simulink model "Parafoil_NL_6DoF_with_Guidance"  (R2019a)
settings: Solver=VariableStepAuto  StartTime=0.0  StopTime=400  RelTol=1e-3
values from neighbouring files (symbols this model uses):
  b = 1.8    [Parafoil_init.m]    (also in Parafoil_init_with_guidance.m)
  c = 3    [Nico_PhaseIIController.m]    (also in Parafoil_init.m = 0.75; Parafoil_init_with_guidance.m = 0.75)
  CD_0 = .153    (= 0.153)    [Parafoil_init.m]    (also in Parafoil_init_with_guidance.m)
  CD_a2 = 2.4    [Parafoil_init.m]    (also in Parafoil_init_with_guidance.m)
  CD_db = .043    (= 0.043)    [Parafoil_init.m]    (also in Parafoil_init_with_guidance.m)
  CD_p = .5    (= 0.5)    [Parafoil_init.m]    (also in Parafoil_init_with_guidance.m)
  CL_0 = 0    [Parafoil_init.m]    (also in Parafoil_init_with_guidance.m)
  CL_a = 3.9    [Parafoil_init.m]    (also in Parafoil_init_with_guidance.m)
  CL_a2db = 2.062    [Parafoil_init.m]    (also in Parafoil_init_with_guidance.m)
  CL_a3 = 20    [Parafoil_init.m]    (also in Parafoil_init_with_guidance.m)
  CL_adb = .39    (= 0.39)    [Parafoil_init.m]    (also in Parafoil_init_with_guidance.m)
  Cl_b = .001    (= 0.001)    [Parafoil_init.m]    (also in Parafoil_init_with_guidance.m)
  Cl_da = 0    [Parafoil_init.m]    (also in Parafoil_init_with_guidance.m)
  CL_db = 0    [Parafoil_init.m]    (also in Parafoil_init_with_guidance.m)
  Cl_p = -.1    (= -0.1)    [Parafoil_init.m]    (also in Parafoil_init_with_guidance.m)
  Cl_r = 0    [Parafoil_init.m]    (also in Parafoil_init_with_guidance.m)
  Cm_db = 0    [Parafoil_init.m]    (also in Parafoil_init_with_guidance.m)
  Cm_q = -2.5    [Parafoil_init.m]    (also in Parafoil_init_with_guidance.m)
  Cn_b = .02    (= 0.02)    [Parafoil_init.m]    (also in Parafoil_init_with_guidance.m)
  Cn_da = .005    (= 0.005)    [Parafoil_init.m]    (also in Parafoil_init_with_guidance.m)
  Cn_da2 = 0    [Parafoil_init.m]    (also in Parafoil_init_with_guidance.m)
  Cn_p = 0    [Parafoil_init.m]    (also in Parafoil_init_with_guidance.m)
  Cn_r = -.11    (= -0.11)    [Parafoil_init.m]    (also in Parafoil_init_with_guidance.m)
  CY_b = -1    [Parafoil_init.m]    (also in Parafoil_init_with_guidance.m)
  db = 0.5*(delR+delL)    (= 0.5)    [Parafoil_init.m]    (also in Parafoil_init_with_guidance.m)
  g = 9.81    [Parafoil_init.m]    (also in Parafoil_init_with_guidance.m)
  gamma_0 = -25*pi/180    (= -0.436332312999)    [Parafoil_init.m]    (also in Parafoil_init_with_guidance.m)
  I_AI = diag([.07 .06 .046])    [Parafoil_init.m]    (also in Parafoil_init_with_guidance.m)
  I_AM = diag([.05 .35 1.85])    [Parafoil_init.m]    (also in Parafoil_init_with_guidance.m)
  I_B = [Ixx Ixy Ixz ... (first row only)    [Parafoil_init.m]    (also in Parafoil_init_with_guidance.m)
  Kd = 0.001    [ARES_GNC_V006_2D.m]    (also in ARES_GNC_V009_2D.m; ARES_GNC_V009_2D_MultiPLot.m; Nico_PhaseIIController.m = 0.5; Parafoil_init_with_guidance.m = 0)
  Ki = 0.003    [ARES_GNC_V006_2D.m]    (also in ARES_GNC_V009_2D.m; ARES_GNC_V009_2D_MultiPLot.m; Nico_PhaseIIController.m = 0.1; Parafoil_init_with_guidance.m = 0.0009)
  Kp = 0.90    (= 0.9)    [ARES_GNC_V006_2D.m]    (also in ARES_GNC_V009_2D.m = 0.05; ARES_GNC_V009_2D_MultiPLot.m = 0.05; Nico_PhaseIIController.m; Parafoil_init_with_guidance.m = 1)
  m = 2.7    [Parafoil_init.m]    (also in Parafoil_init_with_guidance.m)
  p_h = [30;25;0]    [Parafoil_init_with_guidance.m]
  phi_0 = 0*pi/180    (= 0)    [Parafoil_init.m]    (also in Parafoil_init_with_guidance.m)
  psi_0 = 0    [Parafoil_init.m]    (also in Parafoil_init_with_guidance.m)
  r_cg2c = [.5;0;-4]    [Parafoil_init.m]    (also in Parafoil_init_with_guidance.m)
  r_cg2p = [-2; 0; 1]    [Parafoil_init.m]    (also in Parafoil_init_with_guidance.m)
  rho = 1.3    [Parafoil_init.m]    (also in Parafoil_init_with_guidance.m)
  S_rcg2c = [0 -r_cg2c(3) r_cg2c(2) ... (first row only)    [Parafoil_init.m]    (also in Parafoil_init_with_guidance.m)
  Sc = b*c    (= 1.35)    [Parafoil_init.m]    (also in Parafoil_init_with_guidance.m)
  Sp = .01    (= 0.01)    [Parafoil_init.m]    (also in Parafoil_init_with_guidance.m)
  theta_0 = 0*pi/180    (= 0)    [Parafoil_init.m]    (also in Parafoil_init_with_guidance.m)
  v_0 = [7.135; 0; 4.222]    [Parafoil_init.m]    (also in Parafoil_init_with_guidance.m)
  Vw_x = 0    [Parafoil_init.m]    (also in Parafoil_init_with_guidance.m)
  Vw_y = 0    [Parafoil_init.m]    (also in Parafoil_init_with_guidance.m)
  Vw_z = 0    [Parafoil_init.m]    (also in Parafoil_init_with_guidance.m)
  w_0 = [0;0;0]    [Parafoil_init.m]    (also in Parafoil_init_with_guidance.m)
libraries: vrlib x7, simulink x1
settings Model: Creator=chengl2  LastModifiedBy=curryn

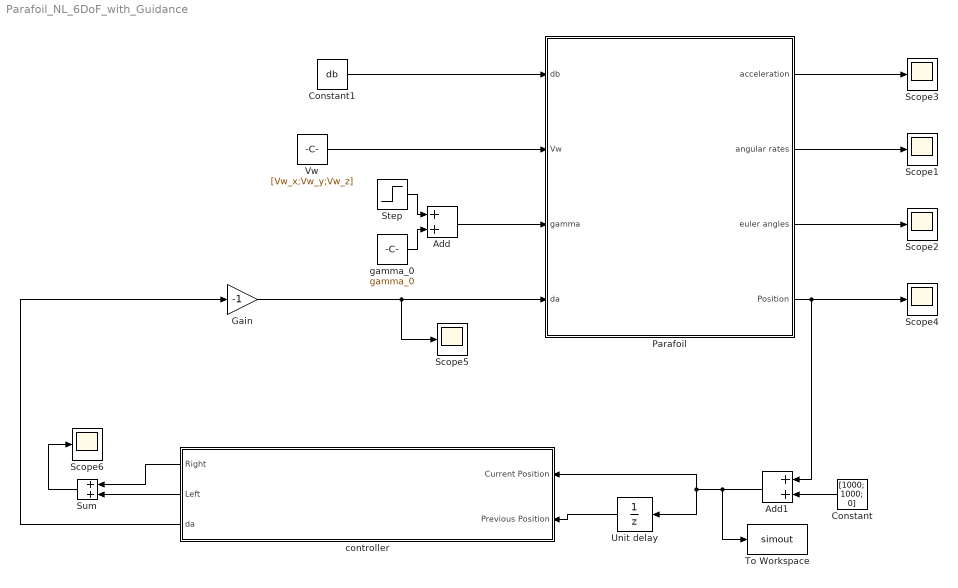
== system Parafoil_NL_6DoF_with_Guidance ==
  Add : Sum
  Add1 : Sum
  Constant : Constant  Value=[1000; 1000; 0]
  Constant1 : Constant  Value=db
  Gain : Gain  Gain=-1
  Parafoil : Subsystem
  Scope{1..6} (6 alike) : Scope
  Step : Step  Time=10  After=0*pi/180  SampleTime=0
  Sum : Sum
  To Workspace : ToWorkspace  VariableName=simout  SaveFormat=Timeseries  SampleTime=-1
  Unit delay : UnitDelay  SampleTime=-1  HasFrameUpgradeWarning=on
  Vw : Constant  Value=[Vw_x;Vw_y;Vw_z]  VectorParams1D=off
  controller : Subsystem
  gamma_0 : Constant  Value=gamma_0
  wires:
  gamma_0/1 -> Add/2
  Step/1 -> Add/1
  Vw/1 -> Parafoil/2(Vw)
  Add/1 -> Parafoil/3(gamma)
  Parafoil/1(acceleration) -> Scope3/1
  Parafoil/2(angular rates) -> Scope1/1
  Parafoil/3(euler angles) -> Scope2/1
  Parafoil/4(Position) -> Add1/1, Scope4/1
  Unit delay/1 -> controller/2(Previous Position)
  Add1/1 -> To Workspace/1, controller/1(Current Position), Unit delay/1
  Constant/1 -> Add1/2
  Gain/1 -> Scope5/1, Parafoil/4(da)
  Constant1/1 -> Parafoil/1(db)
  controller/1(Right) -> Sum/1
  controller/2(Left) -> Sum/2
  controller/3(da) -> Gain/1
  Sum/1 -> Scope6/1

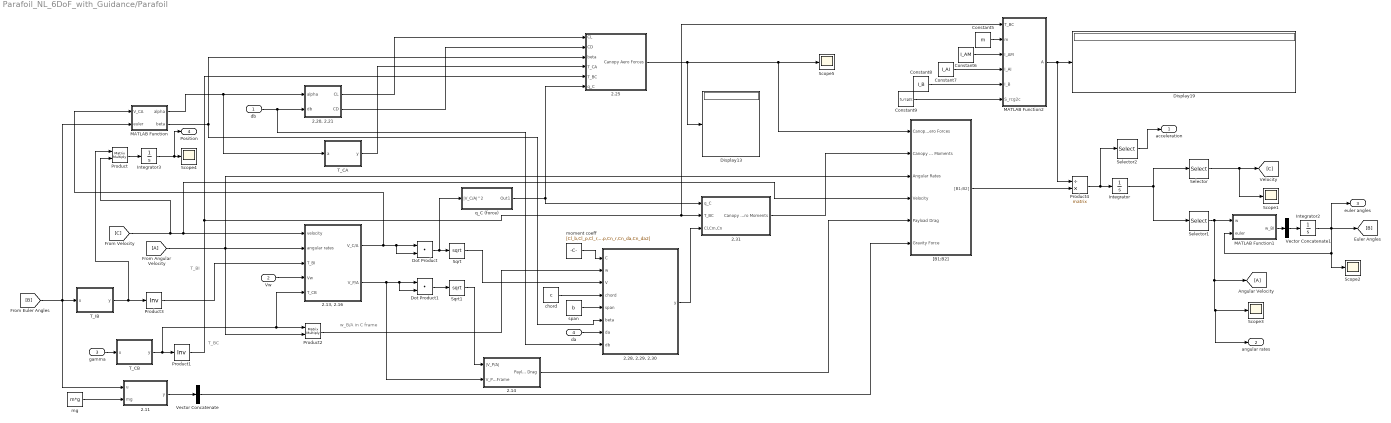
== system Parafoil_NL_6DoF_with_Guidance/Parafoil ==
  note: w_B/A in C frame
  note: T_BC
  note: T_BI
  db : Inport
  Vw : Inport  Port=2
  gamma : Inport  Port=3
  da : Inport  Port=4
  2.11 : MATLAB Function  TreatAsAtomicUnit=on
  "2.13, 2.16" : Subsystem
  2.14 : Subsystem
  "2.20, 2.21 " : Subsystem
  2.25 : Subsystem
  "2.28, 2.29, 2.30" : MATLAB Function  TreatAsAtomicUnit=on
  2.31 : Subsystem
  Constant5 : Constant  Value=m
  Constant6 : Constant  Value=I_AM
  Constant7 : Constant  Value=I_AI
  Constant8 : Constant  Value=I_B
  Constant9 : Constant  Value=S_rcg2c
  Display13 : Display
  Display19 : Display
  Dot Product : DotProduct  InputSameDT=on  OutDataTypeStr=Inherit: Inherit via internal rule
  Dot Product1 : DotProduct  InputSameDT=on  OutDataTypeStr=Inherit: Inherit via internal rule
  Integrator : Integrator  InitialCondition=[v_0;w_0]
  Integrator2 : Integrator  InitialCondition=[phi_0;theta_0;psi_0]
  Integrator3 : Integrator
  MATLAB Function : MATLAB Function  TreatAsAtomicUnit=on
  MATLAB Function1 : MATLAB Function  TreatAsAtomicUnit=on
  MATLAB Function2 : MATLAB Function  TreatAsAtomicUnit=on
  Product : Product  Multiplication=Matrix(*)
  Product1 : Product  Inputs=/  Multiplication=Matrix(*)
  Product2 : Product  Multiplication=Matrix(*)
  Product3 : Product  Inputs=/  Multiplication=Matrix(*)
  Product4 : Product  Inputs=/*  Multiplication=Matrix(*)
  Scope{1..5} (5 alike) : Scope
  Selector : Selector  InputPortWidth=6  IndexOptions=Index vector (dialog)  Indices=[1:3]  OutputSizes=1
  Selector1 : Selector  InputPortWidth=6  IndexOptions=Index vector (dialog)  Indices=[4:6]  OutputSizes=1
  Selector2 : Selector  InputPortWidth=6  IndexOptions=Index vector (dialog)  Indices=[1:3]  OutputSizes=1
  Sqrt : Sqrt  SaturateOnIntegerOverflow=on
  Sqrt1 : Sqrt  SaturateOnIntegerOverflow=on
  T_CA : MATLAB Function  TreatAsAtomicUnit=on
  T_CB : MATLAB Function  TreatAsAtomicUnit=on
  T_IB : MATLAB Function  TreatAsAtomicUnit=on
  Vector Concatenate : Concatenate  NumInputs=1  Mode=Multidimensional array
  Vector Concatenate1 : Concatenate  NumInputs=1  Mode=Multidimensional array
  "[B1;B2]" : Subsystem
  chord : Constant  Value=c
  mg : Constant  Value=m*g
  moment coeff : Constant  Value=[Cl_b,Cl_p,Cl_r,Cl_da,Cm_q,Cm_db,Cn_b,Cn_p,Cn_r,Cn_da,Cn_da2]
  q_C (force) : Subsystem
  span : Constant  Value=b
  acceleration : Outport
  angular rates : Outport  Port=2
  euler angles : Outport  Port=3
  Position : Outport  Port=4
  wires:
  Selector1/1 -> MATLAB Function1/1(w), [A], angular rates/1, Scope3/1
  Sqrt/1 -> "2.28, 2.29, 2.30"/3(V)
  db/1 -> "2.28, 2.29, 2.30"/8(db), "2.20, 2.21 "/2(db)
  "2.28, 2.29, 2.30"/1(y) -> 2.31/3(Cl,Cm,Cn)
  Constant5/1 -> MATLAB Function2/2(m)
  moment coeff/1 -> "2.28, 2.29, 2.30"/1(C)
  [C] -> Product/2, "[B1;B2]"/4(Velocity), "2.13, 2.16"/1(velocity)
  [A] -> "[B1;B2]"/3(Angular Rates), Product2/2, "2.13, 2.16"/2(angular rates)
  Constant6/1 -> MATLAB Function2/3(I_AM)
  Selector/1 -> Scope1/1, [C]
  T_IB/1(y) -> Product3/1, Product/1
  MATLAB Function1/1(w_BI) -> Vector Concatenate1/1
  MATLAB Function2/1(A) -> Product4/1, Display19/1
  Product/1 -> Integrator3/1
  Product4/1 -> Selector2/1, Integrator/1
  "2.13, 2.16"/1(V_C/A) -> MATLAB Function/1(V_CA), Dot Product/2, Dot Product/1
  Constant7/1 -> MATLAB Function2/4(I_AI)
  Product3/1 -> "2.13, 2.16"/3(T_BI)
  MATLAB Function/1(alpha) -> "2.20, 2.21 "/1(alpha), T_CA/1(a)
  mg/1 -> 2.11/2(mg)
  Integrator2/1 -> euler angles/1, [B], MATLAB Function1/2(euler), Scope2/1
  Product2/1 -> "2.28, 2.29, 2.30"/2(w)
  2.25/1(Canopy Aero Forces) -> Display13/1, "[B1;B2]"/1(Canopy Aero Forces), Scope5/1
  q_C (force)/1(Out1) -> 2.25/6(q_C), 2.31/1(q_C)
  "2.20, 2.21 "/2(CD) -> 2.25/2(CD)
  Dot Product1/1 -> Sqrt1/1
  Product1/1 -> 2.25/5(T_BC), MATLAB Function2/1(T_BC), 2.31/2(T_BC)
  Sqrt1/1 -> 2.14/1(|V_P/A|)
  Vector Concatenate1/1 -> Integrator2/1
  "2.20, 2.21 "/1(CL) -> 2.25/1(CL)
  2.11/1(y) -> Vector Concatenate/1
  2.14/1(Payload Drag) -> "[B1;B2]"/5(Payload Drag)
  span/1 -> "2.28, 2.29, 2.30"/5(span)
  T_CA/1(y) -> 2.25/4(T_CA)
  Vector Concatenate/1 -> "[B1;B2]"/6(Gravity Force)
  chord/1 -> "2.28, 2.29, 2.30"/4(chord)
  MATLAB Function/2(beta) -> 2.25/3(beta), "2.28, 2.29, 2.30"/6(beta)
  Integrator/1 -> Selector1/1, Selector/1
  gamma/1 -> T_CB/1(u)
  T_CB/1(y) -> "2.13, 2.16"/5(T_CB), Product2/1, Product1/1
  "[B1;B2]"/1("[B1;B2]") -> Product4/2
  [B] -> MATLAB Function/2(euler), T_IB/1(u), 2.11/1(u)
  da/1 -> "2.28, 2.29, 2.30"/7(da)
  Integrator3/1 -> Position/1, Scope4/1
  Constant8/1 -> MATLAB Function2/5(I_B)
  "2.13, 2.16"/2(V_P/A) -> 2.14/2(V_P/A Body Frame), Dot Product1/2, Dot Product1/1
  2.31/1(Canopy Aero Moments) -> "[B1;B2]"/2(Canopy Aero Moments)
  Constant9/1 -> MATLAB Function2/6(S_rcg2c)
  Dot Product/1 -> q_C (force)/1(|V_C/A|^2), Sqrt/1
  Vw/1 -> "2.13, 2.16"/4(Vw)
  Selector2/1 -> acceleration/1

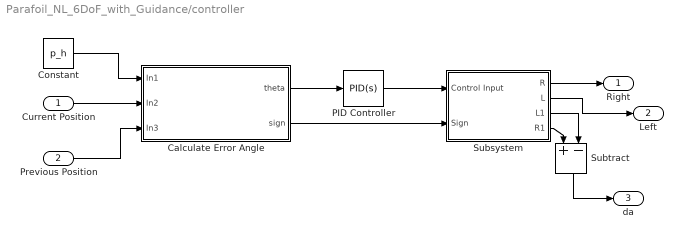
== system Parafoil_NL_6DoF_with_Guidance/controller ==
  Current Position : Inport
  Previous Position : Inport  Port=2
  Calculate Error Angle : Subsystem
  Constant : Constant  Value=p_h
  PID Controller : simulink/Continuous/PID Controller  Controller=PID  Form=Parallel  TimeDomain=Continuous-time  SampleTime=-1  IntegratorMethod=Forward Euler  FilterMethod=Forward Euler  ControllerParametersSource=internal  P=Kp  I=Ki  D=Kd  UseFilter=on  N=100  TunerSelectOption=Transfer Function Based (PID Tuner App)  InitialConditionSource=internal  InitialConditionForIntegrator=0  InitialConditionForFilter=0  DifferentiatorICPrevScaledInput=0  ExternalReset=none  TrackingMode=off  Kt=1  LimitOutput=off  UpperSaturationLimit=inf  LowerSaturationLimit=-inf  LinearizeAsGain=on  AntiWindupMode=none  Kb=1  POutMin=[]  POutMax=[]  IOutMin=[]  IOutMax=[]  DOutMin=[]  DOutMax=[]  NOutMin=[]  NOutMax=[]  SumOutMin=[]  SumOutMax=[]  SaturationOutMin=[]  SaturationOutMax=[]  PParamMin=[]  PParamMax=[]  IParamMin=[]  IParamMax=[]  DParamMin=[]  DParamMax=[]  NParamMin=[]  NParamMax=[]  KbParamMin=[]  KbParamMax=[]  KtParamMin=[]  KtParamMax=[]  KbOutMin=[]  KbOutMax=[]  KtOutMin=[]  KtOutMax=[]  IntegratorOutMin=[]  IntegratorOutMax=[]  FilterOutMin=[]  FilterOutMax=[]  SumI1OutMin=[]  SumI1OutMax=[]  SumI2OutMin=[]  SumI2OutMax=[]  SumI3OutMin=[]  SumI3OutMax=[]  SumI4OutMin=[]  SumI4OutMax=[]  SumDOutMin=[]  SumDOutMax=[]  DifferentiatorOutMin=[]  DifferentiatorOutMax=[]  FilterDiffOutCoefMin=[]  FilterDiffOutCoefMax=[]  ReciprocalOutMin=[]  ReciprocalOutMax=[]  SumDenOutMin=[]  SumDenOutMax=[]  SumNumOutMin=[]  SumNumOutMax=[]  DivideOutMin=[]  DivideOutMax=[]  IntegratorContinuousStateAttributes=''  IntegratorStateMustResolveToSignalObject=off  IntegratorRTWStateStorageClass=Auto  FilterContinuousStateAttributes=''  FilterStateMustResolveToSignalObject=off  FilterRTWStateStorageClass=Auto  ParallelPVariant=InternalParameters  IdealPVariant=Disabled  IVariant=InternalParameters  DVariant=InternalParameters  IntegratorVariant=Continuous  SatVariant=Disabled  AWVariant=Passthrough  PCopyVariant=Disabled  TRVariant=Disabled  FdbkBlocksVariant=Forward  IdealPFdbkVariant=Disabled  SatFdbkVariant=Disabled  DerivativeFilterVariant=ContFilter  NVariant=InternalParameters  NCopyVariant=Disabled  FilterICVariant=InternalICsFilter  IntegratorICVariant=InternalICs  ExternalResetVariant=Disabled  TRSumVariant=Passthrough  SumFdbkVariant=Disabled  SumVariant=Sum_PID
  Subsystem : Subsystem
  Subtract : Sum  Inputs=+-
  Right : Outport
  Left : Outport  Port=2
  da : Outport  Port=3
  wires:
  Constant/1 -> Calculate Error Angle/1(In1)
  Current Position/1 -> Calculate Error Angle/2(In2)
  Previous Position/1 -> Calculate Error Angle/3(In3)
  Calculate Error Angle/1(theta) -> PID Controller/1
  PID Controller/1 -> Subsystem/1(Control Input)
  Calculate Error Angle/2(sign) -> Subsystem/2(Sign)
  Subsystem/1(R) -> Right/1
  Subsystem/2(L) -> Left/1
  Subsystem/3(L1) -> Subtract/2
  Subsystem/4(R1) -> Subtract/1
  Subtract/1 -> da/1

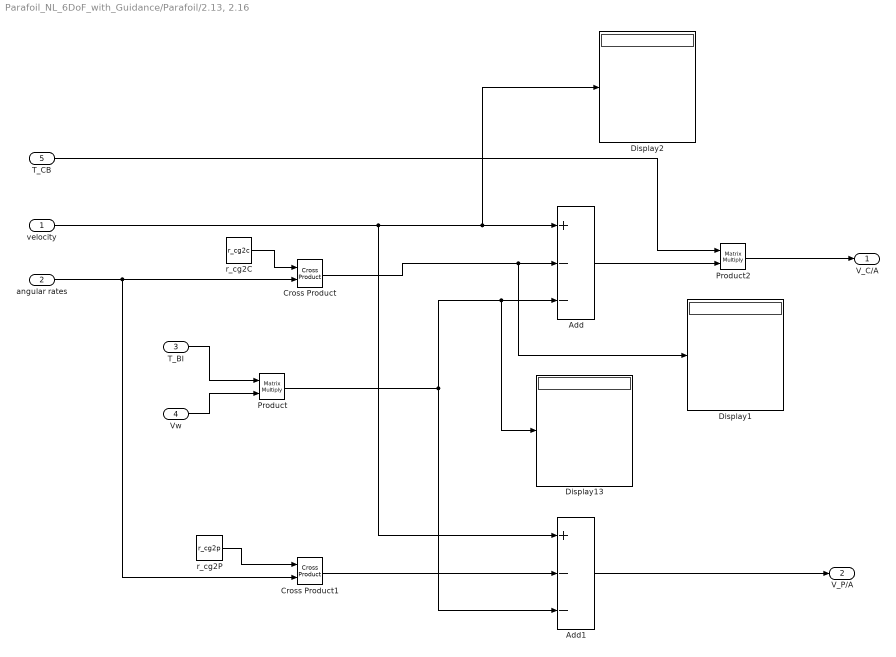
== system Parafoil_NL_6DoF_with_Guidance/Parafoil/2.13, 2.16 ==
  velocity : Inport
  angular rates : Inport  Port=2
  T_BI : Inport  Port=3
  Vw : Inport  Port=4
  T_CB : Inport  Port=5
  Add : Sum  Inputs=+--
  Add1 : Sum  Inputs=+--
  Cross Product : vrlib/Utilities/Cross Product
      settings: SourceProductName=Simulink
  Cross Product1 : vrlib/Utilities/Cross Product
      settings: SourceProductName=Simulink
  Display1 : Display
  Display13 : Display
  Display2 : Display
  Product : Product  Multiplication=Matrix(*)
  Product2 : Product  Multiplication=Matrix(*)
  r_cg2C : Constant  Value=r_cg2c  VectorParams1D=off
  r_cg2P : Constant  Value=r_cg2p  VectorParams1D=off
  V_C/A : Outport
  V_P/A : Outport  Port=2
  wires:
  Vw/1 -> Product/2
  T_BI/1 -> Product/1
  Product2/1 -> V_C/A/1
  angular rates/1 -> Cross Product/2, Cross Product1/2
  velocity/1 -> Add1/1, Display2/1, Add/1
  Cross Product1/1 -> Add1/2
  Product/1 -> Add1/3, Display13/1, Add/3
  Add1/1 -> V_P/A/1
  r_cg2P/1 -> Cross Product1/1
  r_cg2C/1 -> Cross Product/1
  Add/1 -> Product2/2
  T_CB/1 -> Product2/1
  Cross Product/1 -> Display1/1, Add/2

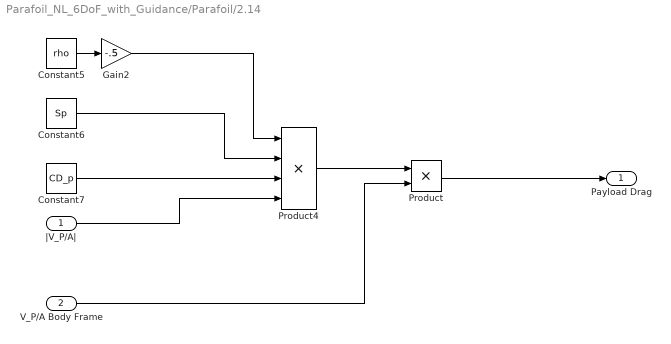
== system Parafoil_NL_6DoF_with_Guidance/Parafoil/2.14 ==
  |V_P/A| : Inport
  V_P/A Body Frame : Inport  Port=2
  Constant5 : Constant  Value=rho
  Constant6 : Constant  Value=Sp
  Constant7 : Constant  Value=CD_p
  Gain2 : Gain  Gain=-.5
  Product : Product
  Product4 : Product  Inputs=4
  Payload Drag : Outport
  wires:
  Constant6/1 -> Product4/2
  Constant7/1 -> Product4/3
  |V_P/A|/1 -> Product4/4
  Gain2/1 -> Product4/1
  Constant5/1 -> Gain2/1
  Product4/1 -> Product/1
  V_P/A Body Frame/1 -> Product/2
  Product/1 -> Payload Drag/1

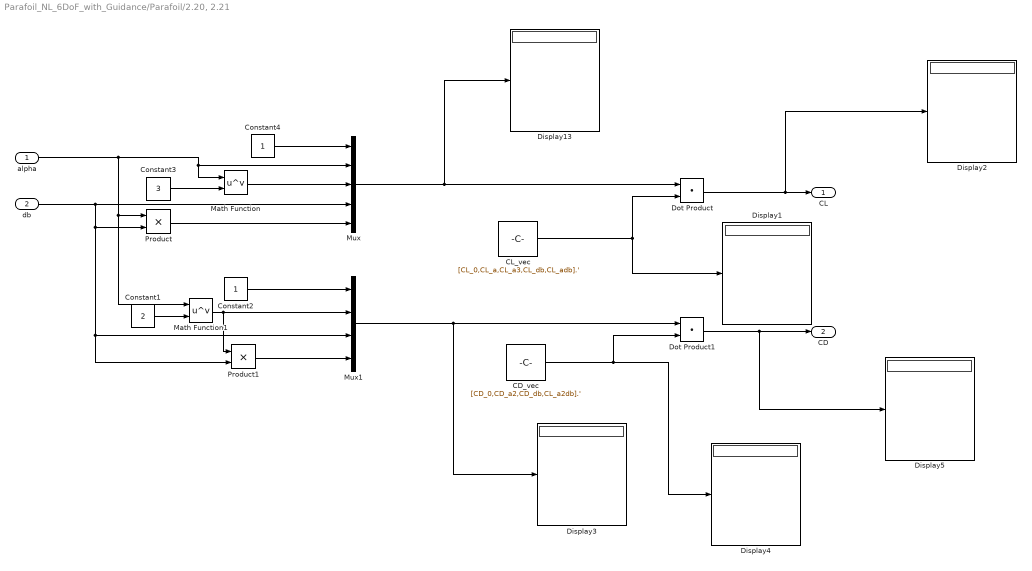
== system Parafoil_NL_6DoF_with_Guidance/Parafoil/2.20, 2.21  ==
  alpha : Inport
  db : Inport  Port=2
  CD_vec : Constant  Value=[CD_0,CD_a2,CD_db,CL_a2db].'
  CL_vec : Constant  Value=[CL_0,CL_a,CL_a3,CL_db,CL_adb].'
  Constant1 : Constant  Value=2
  Constant2 : Constant
  Constant3 : Constant  Value=3
  Constant4 : Constant
  Display{1..5,13} (6 alike) : Display
  Dot Product : DotProduct  InputSameDT=on  OutDataTypeStr=Inherit: Inherit via internal rule
  Dot Product1 : DotProduct  InputSameDT=on  OutDataTypeStr=Inherit: Inherit via internal rule
  Math Function : Math  Operator=pow  SaturateOnIntegerOverflow=on
  Math Function1 : Math  Operator=pow  SaturateOnIntegerOverflow=on
  Mux : Mux  Inputs=5
  Mux1 : Mux
  Product : Product
  Product1 : Product
  CL : Outport
  CD : Outport  Port=2
  wires:
  Math Function/1 -> Mux/3
  Product/1 -> Mux/5
  Mux/1 -> Display13/1, Dot Product/1
  db/1 -> Mux1/3, Product1/2, Product/2, Mux/4
  CL_vec/1 -> Display1/1, Dot Product/2
  alpha/1 -> Product/1, Math Function1/1, Math Function/1, Mux/2
  Dot Product/1 -> Display2/1, CL/1
  Constant4/1 -> Mux/1
  Constant3/1 -> Math Function/2
  Constant1/1 -> Math Function1/2
  Constant2/1 -> Mux1/1
  Math Function1/1 -> Product1/1, Mux1/2
  Product1/1 -> Mux1/4
  CD_vec/1 -> Display4/1, Dot Product1/2
  Dot Product1/1 -> Display5/1, CD/1
  Mux1/1 -> Display3/1, Dot Product1/1

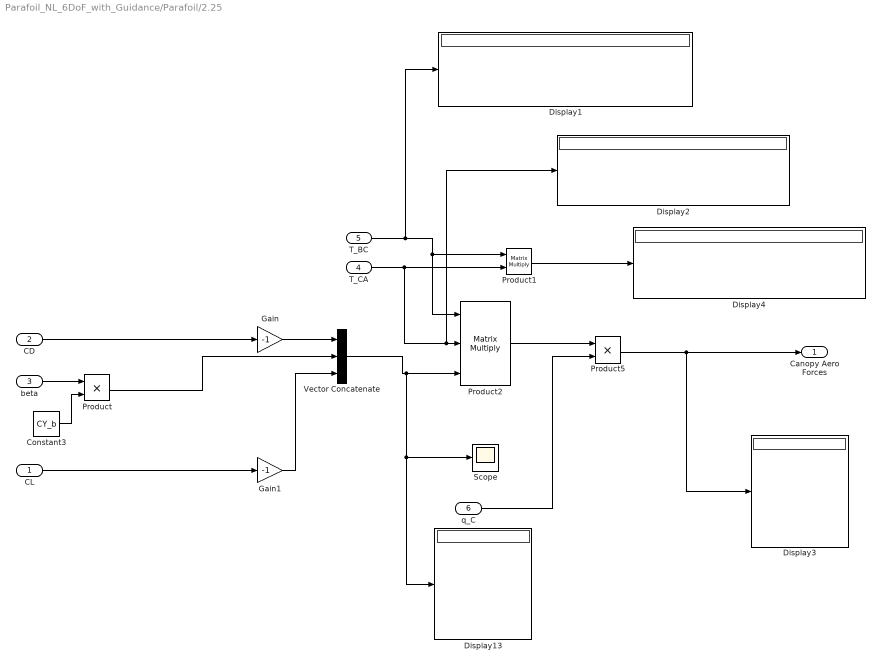
== system Parafoil_NL_6DoF_with_Guidance/Parafoil/2.25 ==
  CL : Inport
  CD : Inport  Port=2
  beta : Inport  Port=3
  T_CA : Inport  Port=4
  T_BC : Inport  Port=5
  q_C : Inport  Port=6
  Constant3 : Constant  Value=CY_b
  Display{1..4,13} (5 alike) : Display
  Gain : Gain  Gain=-1
  Gain1 : Gain  Gain=-1
  Product : Product
  Product1 : Product  Multiplication=Matrix(*)
  Product2 : Product  Inputs=3  Multiplication=Matrix(*)
  Product5 : Product
  Scope : Scope
  Vector Concatenate : Concatenate  NumInputs=3  Mode=Multidimensional array
  Canopy Aero Forces : Outport
  wires:
  T_BC/1 -> Display1/1, Product1/1, Product2/1
  Gain/1 -> Vector Concatenate/1
  Vector Concatenate/1 -> Scope/1, Display13/1, Product2/3
  Product2/1 -> Product5/1
  Product/1 -> Vector Concatenate/2
  beta/1 -> Product/1
  Constant3/1 -> Product/2
  Gain1/1 -> Vector Concatenate/3
  Product5/1 -> Display3/1, Canopy Aero Forces/1
  T_CA/1 -> Product1/2, Display2/1, Product2/2
  q_C/1 -> Product5/2
  CD/1 -> Gain/1
  CL/1 -> Gain1/1
  Product1/1 -> Display4/1

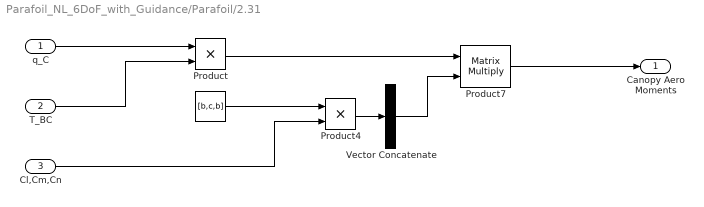
== system Parafoil_NL_6DoF_with_Guidance/Parafoil/2.31 ==
  q_C : Inport
  T_BC : Inport  Port=2
  Cl,Cm,Cn : Inport  Port=3
  " " : Constant  Value=[b,c,b]
  Product : Product
  Product4 : Product
  Product7 : Product  Multiplication=Matrix(*)
  Vector Concatenate : Concatenate  NumInputs=1  Mode=Multidimensional array
  Canopy Aero Moments : Outport
  wires:
  Product7/1 -> Canopy Aero Moments/1
  " "/1 -> Product4/1
  Product4/1 -> Vector Concatenate/1
  Vector Concatenate/1 -> Product7/2
  Cl,Cm,Cn/1 -> Product4/2
  Product/1 -> Product7/1
  T_BC/1 -> Product/2
  q_C/1 -> Product/1

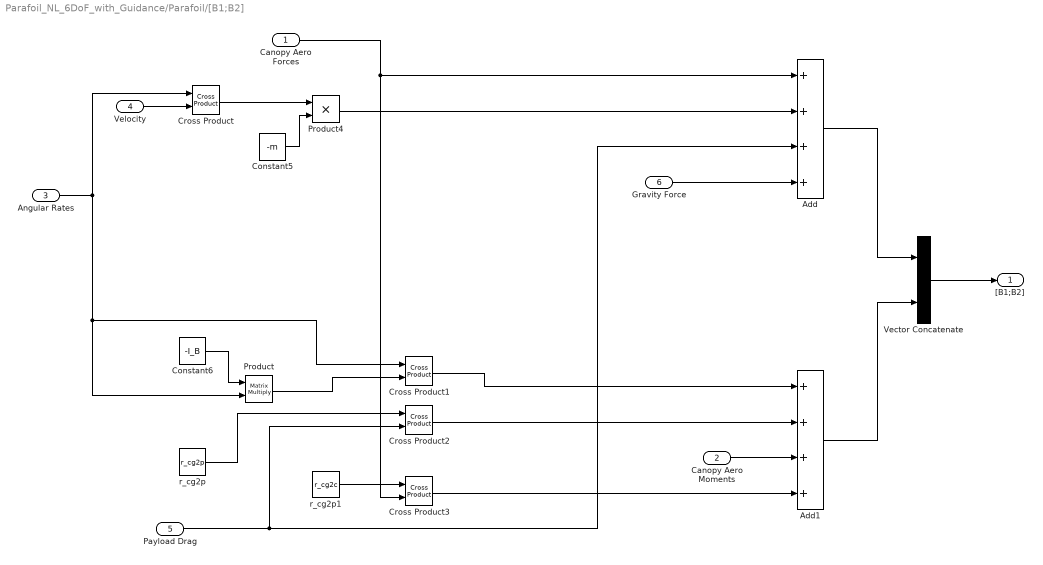
== system Parafoil_NL_6DoF_with_Guidance/Parafoil/[B1;B2] ==
  Canopy Aero Forces : Inport
  Canopy Aero Moments : Inport  Port=2
  Angular Rates : Inport  Port=3
  Velocity : Inport  Port=4
  Payload Drag : Inport  Port=5
  Gravity Force : Inport  Port=6
  Add : Sum  Inputs=++++
  Add1 : Sum  Inputs=++++
  Constant5 : Constant  Value=-m
  Constant6 : Constant  Value=-I_B
  Cross Product{,1..3} (4 alike) : vrlib/Utilities/Cross Product
      settings: SourceProductName=Simulink
  Product : Product  Multiplication=Matrix(*)
  Product4 : Product
  Vector Concatenate : Concatenate
  r_cg2p : Constant  Value=r_cg2p  VectorParams1D=off
  r_cg2p1 : Constant  Value=r_cg2c  VectorParams1D=off
  "[B1;B2]" : Outport
  wires:
  Cross Product3/1 -> Add1/4
  r_cg2p/1 -> Cross Product2/1
  Cross Product1/1 -> Add1/1
  Canopy Aero Forces/1 -> Cross Product3/2, Add/1
  Angular Rates/1 -> Cross Product/1, Cross Product1/1, Product/2
  Payload Drag/1 -> Add/3, Cross Product2/2
  Product/1 -> Cross Product1/2
  Constant5/1 -> Product4/2
  Product4/1 -> Add/2
  Cross Product2/1 -> Add1/2
  Constant6/1 -> Product/1
  Cross Product/1 -> Product4/1
  Vector Concatenate/1 -> "[B1;B2]"/1
  Gravity Force/1 -> Add/4
  Add1/1 -> Vector Concatenate/2
  Add/1 -> Vector Concatenate/1
  Velocity/1 -> Cross Product/2
  Canopy Aero Moments/1 -> Add1/3
  r_cg2p1/1 -> Cross Product3/1

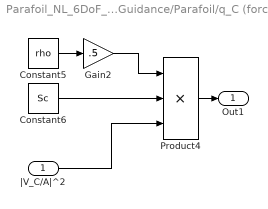
== system Parafoil_NL_6DoF_with_Guidance/Parafoil/q_C (force) ==
  |V_C/A|^2 : Inport
  Constant5 : Constant  Value=rho
  Constant6 : Constant  Value=Sc
  Gain2 : Gain  Gain=.5
  Product4 : Product  Inputs=3
  Out1 : Outport
  wires:
  Gain2/1 -> Product4/1
  Constant6/1 -> Product4/2
  Constant5/1 -> Gain2/1
  Product4/1 -> Out1/1
  |V_C/A|^2/1 -> Product4/3

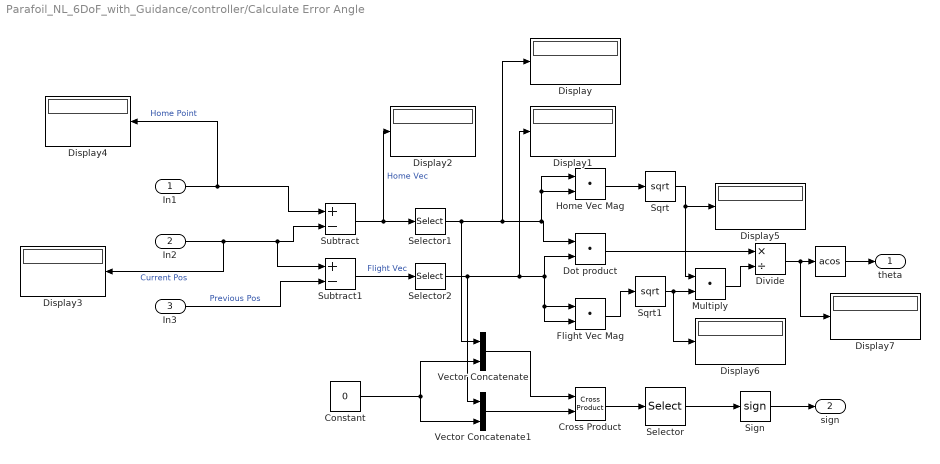
== system Parafoil_NL_6DoF_with_Guidance/controller/Calculate Error Angle ==
  In1 : Inport
  In2 : Inport  Port=2
  In3 : Inport  Port=3
  " " : Trigonometry  Operator=acos
  Constant : Constant  Value=0
  Cross Product : vrlib/Utilities/Cross Product
      settings: SourceProductName=Simulink
  Display{,1..7} (8 alike) : Display
  Divide : Product  Inputs=*/
  Dot product : DotProduct  InputSameDT=on  OutDataTypeStr=Inherit: Inherit via internal rule
  Flight Vec Mag : DotProduct  InputSameDT=on  OutDataTypeStr=Inherit: Inherit via internal rule
  Home Vec Mag : DotProduct  InputSameDT=on  OutDataTypeStr=Inherit: Inherit via internal rule
  Multiply : DotProduct  InputSameDT=on  OutDataTypeStr=Inherit: Inherit via internal rule
  Selector : Selector  InputPortWidth=3  IndexOptions=Index vector (dialog)  Indices=3  OutputSizes=1
  Selector1 : Selector  InputPortWidth=3  IndexOptions=Index vector (dialog)  Indices=[1, 2]  OutputSizes=1
  Selector2 : Selector  InputPortWidth=3  IndexOptions=Index vector (dialog)  Indices=[1, 2]  OutputSizes=1
  Sign : Signum
  Sqrt : Sqrt  SaturateOnIntegerOverflow=on
  Sqrt1 : Sqrt  SaturateOnIntegerOverflow=on
  Subtract : Sum  Inputs=+-
  Subtract1 : Sum  Inputs=+-
  Vector Concatenate : Concatenate
  Vector Concatenate1 : Concatenate
  theta : Outport
  sign : Outport  Port=2
  wires:
  Multiply/1 -> Divide/2
  Subtract1/1 -> Selector2/1  "Flight Vec"
  Dot product/1 -> Divide/1
  Divide/1 -> Display7/1, " "/1
  Home Vec Mag/1 -> Sqrt/1
  Subtract/1 -> Display2/1, Selector1/1  "Home Vec"
  Flight Vec Mag/1 -> Sqrt1/1
  In2/1 -> Display3/1, Subtract1/1, Subtract/2  "Current Pos"
  In1/1 -> Display4/1, Subtract/1  "Home Point"
  In3/1 -> Subtract1/2  "Previous Pos"
  " "/1 -> theta/1
  Sqrt/1 -> Multiply/1, Display5/1
  Sqrt1/1 -> Display6/1, Multiply/2
  Cross Product/1 -> Selector/1
  Selector/1 -> Sign/1
  Sign/1 -> sign/1
  Selector1/1 -> Vector Concatenate/1, Display/1, Home Vec Mag/2, Home Vec Mag/1, Dot product/1
  Selector2/1 -> Vector Concatenate1/1, Display1/1, Flight Vec Mag/2, Flight Vec Mag/1, Dot product/2
  Constant/1 -> Vector Concatenate/2, Vector Concatenate1/2
  Vector Concatenate/1 -> Cross Product/1
  Vector Concatenate1/1 -> Cross Product/2

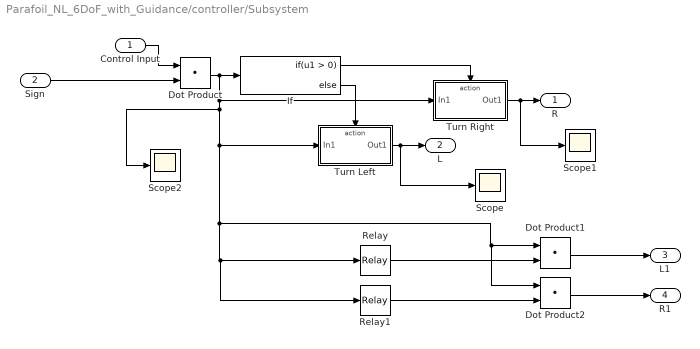
== system Parafoil_NL_6DoF_with_Guidance/controller/Subsystem ==
  Control Input : Inport
  Sign : Inport  Port=2
  Dot Product : DotProduct  InputSameDT=on  OutDataTypeStr=Inherit: Inherit via internal rule
  Dot Product1 : DotProduct  InputSameDT=on  OutDataTypeStr=Inherit: Inherit via internal rule
  Dot Product2 : DotProduct  InputSameDT=on  OutDataTypeStr=Inherit: Inherit via internal rule
  If : If
  Relay : Relay  OnSwitchValue=0.0001  OffSwitchValue=-0.0001  OnOutputValue=0  OffOutputValue=-1
  Relay1 : Relay  OnSwitchValue=0.0001  OffSwitchValue=-0.0001
  Scope : Scope
  Scope1 : Scope
  Scope2 : Scope
  "Turn Left " : Subsystem  TreatAsAtomicUnit=on
  Turn Right : Subsystem  TreatAsAtomicUnit=on
  R : Outport
  L : Outport  Port=2
  L1 : Outport  Port=3
  R1 : Outport  Port=4
  wires:
  Sign/1 -> Dot Product/2
  Turn Right/1(Out1) -> Scope1/1, R/1
  Dot Product/1 -> Scope2/1, Dot Product2/1, Dot Product1/1, Relay1/1, Relay/1, "Turn Left "/1(In1), Turn Right/1(In1), If/1
  If/1 -> Turn Right/Action
  "Turn Left "/1(Out1) -> Scope/1, L/1
  If/2 -> "Turn Left "/Action
  Control Input/1 -> Dot Product/1
  Relay/1 -> Dot Product1/2
  Relay1/1 -> Dot Product2/2
  Dot Product1/1 -> L1/1
  Dot Product2/1 -> R1/1

== system Parafoil_NL_6DoF_with_Guidance/controller/Subsystem/Turn Left  ==
  In1 : Inport
  Action Port : ActionPort  ActionPortLabel=else
  Out1 : Outport
  wires:
  In1/1 -> Out1/1

== system Parafoil_NL_6DoF_with_Guidance/controller/Subsystem/Turn Right ==
  In1 : Inport
  Action Port : ActionPort  ActionPortLabel=if(u1 > 0)
  Out1 : Outport
  wires:
  In1/1 -> Out1/1

== matlab function Parafoil_NL_6DoF_with_Guidance/Parafoil/T_CB ==
  data: u input; y output
function y = T_CB(u)
    % calculates transformation matrix T_CB from gamma in radians
    %goes from body frame to canopy frame R(J_B,gamma)
    
    y = [cos(u) 0 -sin(u)  
        0 1 0
        sin(u) 0 cos(u)];

== matlab function Parafoil_NL_6DoF_with_Guidance/Parafoil/T_IB ==
  data: u input; y output
function y = T_IB(u)
    %calculates transformation matrix T_IB (Body frame to Inertial frame) from Euler angles in radians
    

    y = [cos(u(2))*cos(u(3)),sin(u(1))*sin(u(2))*cos(u(3)) - cos(u(1))*sin(u(3)),cos(u(1))*sin(u(2))*cos(u(3)) + sin(u(1))*sin(u(3))
        cos(u(2))*sin(u(3)),sin(u(1))*sin(u(2))*sin(u(3)) + cos(u(1))*cos(u(3)),cos(u(1))*sin(u(2))*sin(u(3)) - sin(u(1))*cos(u(3))
        -sin(u(2)), sin(u(1))*cos(u(2)), cos(u(1))*cos(u(2))];
%     y = [cos(u(2))*cos(u(3)), cos(u(2))*sin(u(3)), -sin(u(2))
%     sin(u(1))*sin(u(2))*cos(u(3)) - cos(u(1))*sin(u(3)), sin(u(1))*sin(u(2))*sin(u(3)) + cos(u(1))*cos(u(3)), sin(u(1))*cos(u(2))
%     cos(u(1))*sin(u(2))*cos(u(3)) + sin(u(1))*sin(u(3)), cos(u(1))*sin(u(2))*sin(u(3)) - sin(u(1))*cos(u(3)), cos(u(1))*cos(u(2))];

== matlab function Parafoil_NL_6DoF_with_Guidance/Parafoil/2.11 ==
  data: u input; y output; mg input
function y = Eq_2_11(u,mg)
%Calculates gravitational force in the body frame
    
y = mg*[-sin(u(2));sin(u(1))*cos(u(2)); cos(u(1))*cos(u(2))];

== matlab function Parafoil_NL_6DoF_with_Guidance/Parafoil/T_CA ==
  data: a input; y output
function y = T_CA(a)
    % calculates transformation matrix T_CA from alpha in radians
    %goes from aero velocity frame to canopy frame R(J_C,alpha)
    
    y = [cos(a) 0 -sin(a)  
        0 1 0
        sin(a) 0 cos(a)];

== matlab function Parafoil_NL_6DoF_with_Guidance/Parafoil/2.28, 2.29, 2.30 ==
  data: C input; y output; w input; V input; chord input; span input; beta input; da input; db input
function y  = Moment_coeff(C,w,V,chord,span,beta,da,db)
    % Calculates the buildup of aerodynamic moments 
    % from Cacan Eq 2.28,2.29,2.30
    
    p = w(1); q = w(2); r = w(3); %angular velocity wrt to atmospheric winds in the canopy frame
    
    Cl = C(1)*beta + (span/(2*V))*(C(2)*p + C(3)*r) + C(4)*da;
    Cm = (chord/(2*V))*C(5)*q + C(6)*db;
    Cn = C(7)*beta + (span/(2*V))*(C(8)*p + C(9)*r) + C(10)*da + C(11)*da^2;

y = [Cl;Cm;Cn];

== matlab function Parafoil_NL_6DoF_with_Guidance/Parafoil/MATLAB Function ==
  data: V_CA input; alpha output; beta output; euler input
function [alpha,beta] = fcn(V_CA,euler)

alpha = atan2(V_CA(3)/cos(euler(2)),V_CA(1)/cos(euler(2))); 

beta =  asin(V_CA(2)/norm(V_CA));

== matlab function Parafoil_NL_6DoF_with_Guidance/Parafoil/MATLAB Function1 ==
  data: w input; w_BI output; euler input
function w_BI = Eq_2_6(w,euler)
    %Transforms body angular rotation rates (p,q,r) to 
    %Euler derivatives (phi_dot,theta_dot,psi_dot)
    %Note1: Cacan eq 2.6 has the 2nd row 3rd column entry as -sin(theta) 
    %I believe that is a typo in the Cacan dissertation
    %See eq 7.3.19 in mechanics of flight 2nd ed Warren Ed Phillips 
    %Note2: This transformation is not suitable for flight code due to 
    %potential gimabal lock. For use in simulation only. 
    phi = euler(1);theta = euler(2);
   
    w_BI = [1, sin(phi)*tan(theta), cos(phi)*tan(theta)
        0, cos(phi), -sin(theta)
        0, sin(phi)/cos(theta),cos(phi)/cos(theta)]*w;

== matlab function Parafoil_NL_6DoF_with_Guidance/Parafoil/MATLAB Function2 ==
  data: T_BC input; A output; m input; I_AM input; I_AI input; I_B input; S_rcg2c input
function A = fcn(T_BC,m,I_AM,I_AI,I_B,S_rcg2c)
%const = [m,I_AM,I_AI,I_B,S_rcg2c]


A = [m*eye(3,3) + T_BC*I_AM*T_BC.', -T_BC*I_AM*T_BC.'*S_rcg2c
    S_rcg2c*T_BC*I_AM*T_BC.', I_B + T_BC*I_AI*T_BC.' - S_rcg2c*T_BC*I_AM*T_BC.'*S_rcg2c];
